simulink model "Plant_3"  (R2024b)
settings: Solver=FixedStepAuto  StartTime=0.0  StopTime=2  FixedStep=0.02  RelTol=1e-3
PreLoadFcn:
  | addpath("ref_source\")
model workspace (MAT data in the model file):
  Ref_sig_idx = 2
values from neighbouring files (symbols this model uses):
  A = zeros(4, 4)    [Initialise_var_0.m]
  B = zeros(4, 2)    [Initialise_var_0.m]
  C = [1 0 0 0; 0 1 0 0; 0 0 1 0; 0 0 0 1]    [Initialise_var_0.m]    (also in leunberger_obs_1.m = [1 0 0 0; 0 1 0 0]; sfbia.m = [1 0 0 0; 0 1 0 0])
  D = [0 0; 0 0; 0 0; 0 0]    [Initialise_var_0.m]    (also in leunberger_obs_1.m = [0 0;0 0]; sfbia.m = [0 0;0 0])
  G = [G1; G2]    [Initialise_var_0.m]    (also in leunberger_obs_1.m = place(A', C', desired_poles)')
  K = place(A, B, desired_poles)    [leunberger_obs_1.m]    (also in state_feedback.m; state_feedback_0.m; state_feedback_3.m; state_feedback_4.m = lqr(A,B,Q,R))
  K_r_lo = -inv(C*inv(A-B*K)*B)    [leunberger_obs_1.m]
  L1 = 0.095    [Initialise_var_0.m]
  L2 = 0.095    [Initialise_var_0.m]
settings Model: Creator=Sez26  LastModifiedBy=Sez26

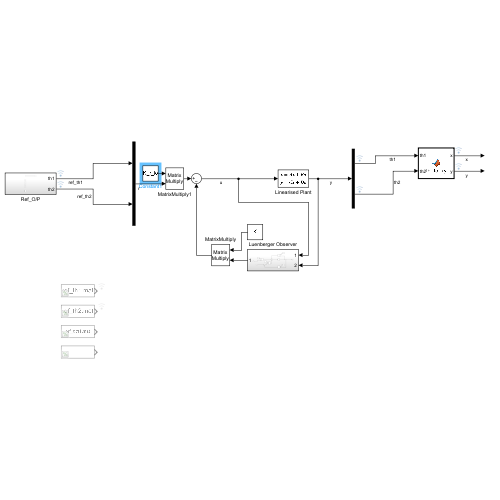
[thumbnail: Simulink's stored preview of the top-level diagram]
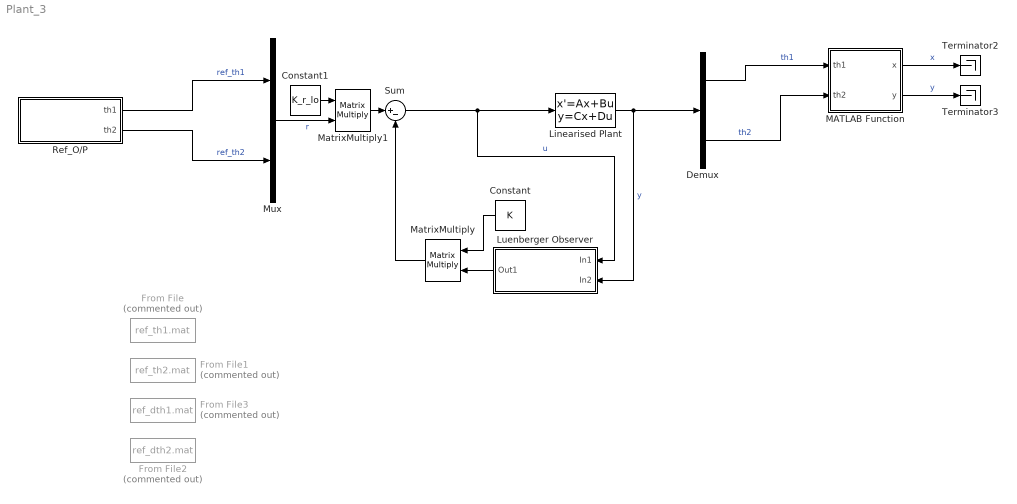
== system Plant_3 ==
  Constant : Constant  Value=K
  Constant1 : Constant  Value=K_r_lo
  Demux : Demux  Outputs=2
  From File : FromFile  Commented=on  FileName=ref_th1.mat  SampleTime=0
  From File1 : FromFile  Commented=on  FileName=ref_th2.mat  SampleTime=0
  From File2 : FromFile  Commented=on  FileName=ref_dth2.mat  SampleTime=0
  From File3 : FromFile  Commented=on  FileName=ref_dth1.mat  SampleTime=0
  Linearised Plant : StateSpace  A=A  B=B  C=C  D=D  InitialCondition=0
  Luenberger Observer : Subsystem
  MATLAB Function : MATLAB Function  TreatAsAtomicUnit=on
  MatrixMultiply : Product  Multiplication=Matrix(*)
  MatrixMultiply1 : Product  Multiplication=Matrix(*)
  Mux : Mux  Inputs=2
  Ref_O/P : Subsystem
  Sum : Sum  Inputs=|+-
  Terminator2 : Terminator
  Terminator3 : Terminator
  wires:
  MATLAB Function/1(x) -> Terminator2/1  "x"
  MATLAB Function/2(y) -> Terminator3/1  "y"
  Demux/2 -> MATLAB Function/2(th2)  "th2"
  Demux/1 -> MATLAB Function/1(th1)  "th1"
  Linearised Plant/1 -> Luenberger Observer/2(In2), Demux/1  "y"
  Ref_O/P/1(th1) -> Mux/1  "ref_th1"
  Ref_O/P/2(th2) -> Mux/2  "ref_th2"
  Luenberger Observer/1(Out1) -> MatrixMultiply/2
  Constant/1 -> MatrixMultiply/1
  Mux/1 -> MatrixMultiply1/2  "r"
  Constant1/1 -> MatrixMultiply1/1
  MatrixMultiply1/1 -> Sum/1
  MatrixMultiply/1 -> Sum/2
  Sum/1 -> Luenberger Observer/1(In1), Linearised Plant/1  "u"

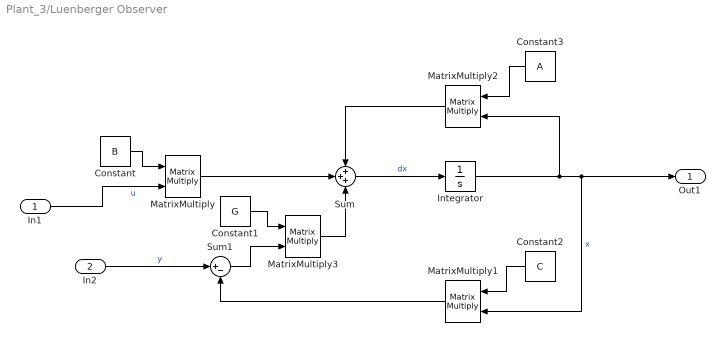
== system Plant_3/Luenberger Observer ==
  In1 : Inport
  In2 : Inport  Port=2
  Constant : Constant  Value=B
  Constant1 : Constant  Value=G
  Constant2 : Constant  Value=C
  Constant3 : Constant  Value=A
  Integrator : Integrator
  MatrixMultiply{,1..3} (4 alike) : Product  Multiplication=Matrix(*)
  Sum : Sum  Inputs=+++
  Sum1 : Sum  Inputs=|+-
  Out1 : Outport
  wires:
  In1/1 -> MatrixMultiply/2  "u"
  Constant/1 -> MatrixMultiply/1
  MatrixMultiply/1 -> Sum/2
  Sum/1 -> Integrator/1  "dx"
  In2/1 -> Sum1/1  "y"
  Integrator/1 -> MatrixMultiply2/2, Out1/1, MatrixMultiply1/2  "x"
  Constant2/1 -> MatrixMultiply1/1
  MatrixMultiply1/1 -> Sum1/2
  Constant1/1 -> MatrixMultiply3/1
  Sum1/1 -> MatrixMultiply3/2
  MatrixMultiply3/1 -> Sum/3
  MatrixMultiply2/1 -> Sum/1
  Constant3/1 -> MatrixMultiply2/1

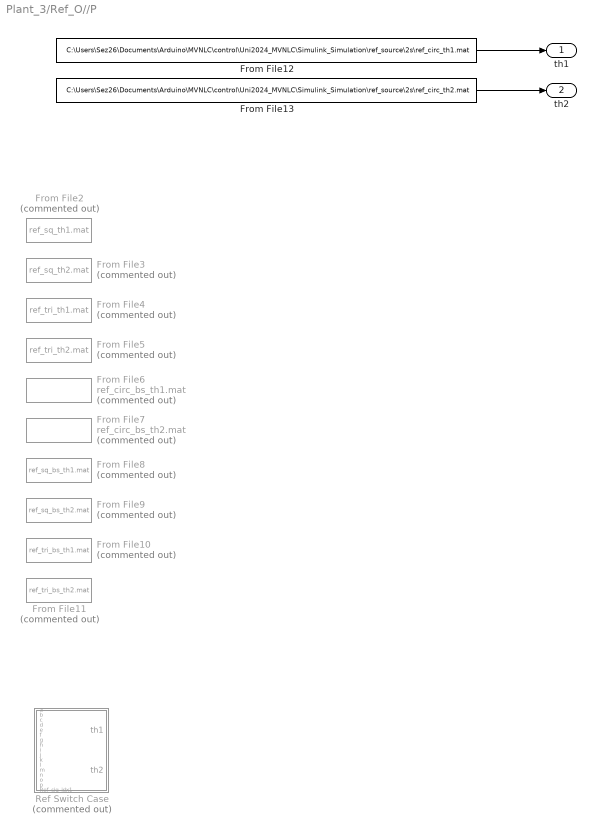
== system Plant_3/Ref_O//P ==
  From File10 : FromFile  Commented=on  FileName=ref_tri_bs_th1.mat  SampleTime=0
  From File11 : FromFile  Commented=on  FileName=ref_tri_bs_th2.mat  SampleTime=0
  From File12 : FromFile  FileName=C:\Users\Sez26\Documents\Arduino\MVNLC\control\Uni2024_MVNLC\Simulink_Simulation\ref_source\2s\ref_circ_th1.mat  SampleTime=0
  From File13 : FromFile  FileName=C:\Users\Sez26\Documents\Arduino\MVNLC\control\Uni2024_MVNLC\Simulink_Simulation\ref_source\2s\ref_circ_th2.mat  SampleTime=0
  From File2 : FromFile  Commented=on  FileName=ref_sq_th1.mat  SampleTime=0
  From File3 : FromFile  Commented=on  FileName=ref_sq_th2.mat  SampleTime=0
  From File4 : FromFile  Commented=on  FileName=ref_tri_th1.mat  SampleTime=0
  From File5 : FromFile  Commented=on  FileName=ref_tri_th2.mat  SampleTime=0
  From File6 : FromFile  Commented=on  FileName=ref_circ_bs_th1.mat  SampleTime=0
  From File7 : FromFile  Commented=on  FileName=ref_circ_bs_th2.mat  SampleTime=0
  From File8 : FromFile  Commented=on  FileName=ref_sq_bs_th1.mat  SampleTime=0
  From File9 : FromFile  Commented=on  FileName=ref_sq_bs_th2.mat  SampleTime=0
  Ref Switch Case : MATLAB Function  Commented=on  TreatAsAtomicUnit=on
  th1 : Outport
  th2 : Outport  Port=2
  wires:
  From File12/1 -> th1/1
  From File13/1 -> th2/1

== matlab function Plant_3/Ref_O//P/Ref Switch Case ==
  data: Ref_sig_idx parameter; a input; b input; c input; d input; e input; f input; g input; h input; i input; j input; k input; l input; m input; n input; o input; p input; Ref_sig_idx1 input; th1 output; th2 output
function [th1, th2] = ref_switch(Ref_sig_idx, a, b, c, d, e, f, g, h, i, j, k, l, m, n, o, p, Ref_sig_idx1)
    if Ref_sig_idx == 0
        % circ base
        th1 = a;
        th2 = b;
    elseif Ref_sig_idx == 1
        % sq base
        th1 = c;
        th2 = d;
    elseif Ref_sig_idx == 2
        % tri base
        th1 = e;
        th2 = f;
    end
    if Ref_sig_idx == 3
        % circ b spline
        th1 = g;
        th2 = h;
    elseif Ref_sig_idx == 4
        % sq b spline
        th1 = i;
        th2 = j;
    elseif Ref_sig_idx == 5
        % tri b spline
        th1 = k;
        th2 = l;
    end
    if Ref_sig_idx == 6
        % sq corner sf
        th1 = m;
        th2 = n;
    elseif Ref_sig_idx == 7
        % tri corner sf
        th1 = o;
        th2 = p;
    else
        % invalid reference choice
        disp('Error invalid reference choice')
        th1 = 0;
        th2 = 0;
    end

== matlab function Plant_3/MATLAB Function ==
  data: x output; th1 input; y output; th2 input; L1 parameter; L2 parameter
function [x,y] = th_to_xy(th1, th2, L1, L2)
    x = L1*cos(deg2rad(th1)) + L2*cos(deg2rad(th2));
    y = L1*sin(deg2rad(th1)) + L2*sin(deg2rad(th2));
